simulink model "DC_motor_Control"  (R2022b)
settings: Solver=VariableStepAuto  StartTime=0.0  StopTime=10.0  RelTol=1e-3
settings Model: Creator=AhmedSamy  LastModifiedBy=AhmedSamy

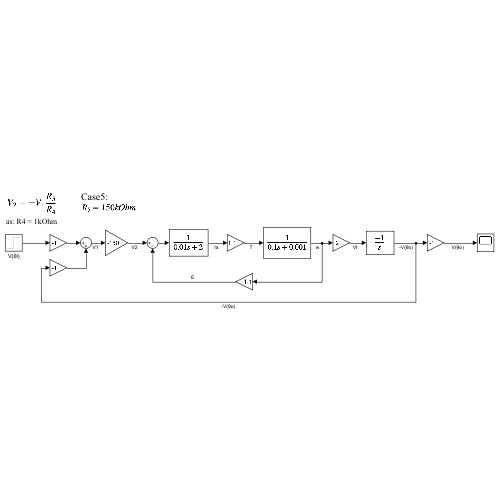
[thumbnail: Simulink's stored preview of the top-level diagram]
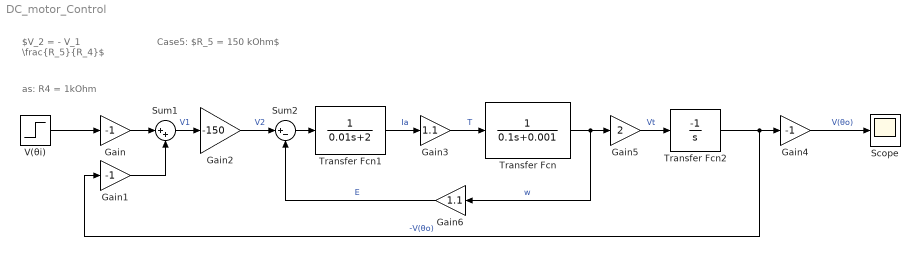
== system DC_motor_Control ==
  note: Case5:
      | $R_5 = 150 kOhm$
  note: $V_2 = - V_1 \frac{R_5}{R_4}$
  note: as: R4 = 1kOhm
  Gain : Gain  Gain=-1
  Gain1 : Gain  Gain=-1
  Gain2 : Gain  Gain=-150
  Gain3 : Gain  Gain=1.1
  Gain4 : Gain  Gain=-1
  Gain5 : Gain  Gain=2
  Gain6 : Gain  Gain=1.1
  Scope : Scope
  Sum1 : Sum  Inputs=|++
  Sum2 : Sum  Inputs=|+-
  Transfer Fcn : TransferFcn  Denominator=[0.1 0.001]
  Transfer Fcn1 : TransferFcn  Denominator=[0.01 2]
  Transfer Fcn2 : TransferFcn  Numerator=[-1]  Denominator=[1 0]
  V(θi) : Step  Time=0  After=10  SampleTime=0
  wires:
  V(θi)/1 -> Gain/1
  Gain/1 -> Sum1/1
  Gain1/1 -> Sum1/2
  Sum1/1 -> Gain2/1  "V1"
  Gain2/1 -> Sum2/1  "V2"
  Sum2/1 -> Transfer Fcn1/1
  Gain6/1 -> Sum2/2  "E"
  Transfer Fcn1/1 -> Gain3/1  "Ia"
  Gain3/1 -> Transfer Fcn/1  "T"
  Gain5/1 -> Transfer Fcn2/1  "Vt"
  Transfer Fcn/1 -> Gain6/1, Gain5/1  "w"
  Transfer Fcn2/1 -> Gain4/1, Gain1/1  "-V(θo)"
  Gain4/1 -> Scope/1  "V(θo)"
